simulink model "burckhardt_tire_model"  (R2022b)
settings: Solver=VariableStepAuto  StartTime=0.0  StopTime=10.0  RelTol=1e-3
values from neighbouring files (symbols this model uses):
  Fz = 3000    [burckhardt_model.m]
  road_type = i    [burckhardt_model.m]
undefined symbols (not defined in the file or in its folder): s
settings Model: Creator=FATMANURATA  LastModifiedBy=FATMANURATA

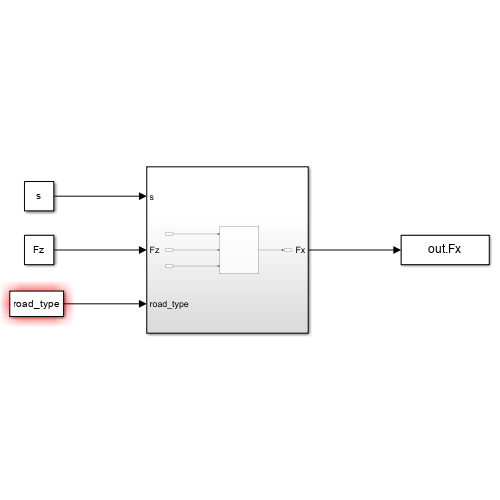
[thumbnail: Simulink's stored preview of the top-level diagram]
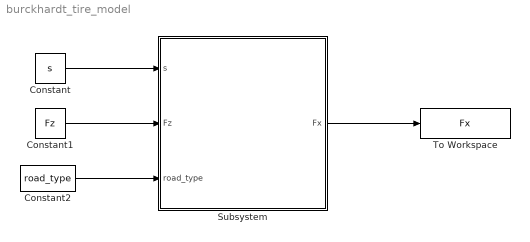
== system burckhardt_tire_model ==
  Constant : Constant  Value=s
  Constant1 : Constant  Value=Fz
  Constant2 : Constant  Value=road_type
  Subsystem : Subsystem
  To Workspace : ToWorkspace  VariableName=Fx  SampleTime=-1
  wires:
  Constant/1 -> Subsystem/1(s)
  Constant1/1 -> Subsystem/2(Fz)
  Constant2/1 -> Subsystem/3(road_type)
  Subsystem/1(Fx) -> To Workspace/1

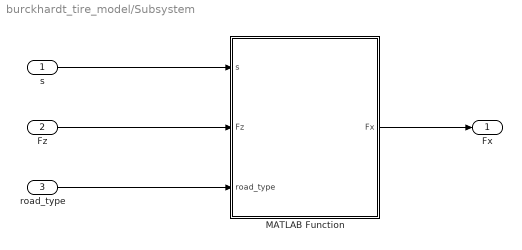
== system burckhardt_tire_model/Subsystem ==
  s : Inport
  Fz : Inport  Port=2
  road_type : Inport  Port=3
  MATLAB Function : MATLAB Function  TreatAsAtomicUnit=on
  Fx : Outport
  wires:
  s/1 -> MATLAB Function/1(s)
  MATLAB Function/1(Fx) -> Fx/1
  Fz/1 -> MATLAB Function/2(Fz)
  road_type/1 -> MATLAB Function/3(road_type)

== matlab function burckhardt_tire_model/Subsystem/MATLAB Function ==
  data: s input; Fx output; Fz input; road_type input
function Fx = fcn(s, Fz, road_type)
   
    % Table:  Burckhardttiremodelparameters.
    

    %      c1       c2        c3
    C = [1.2801, 23.9900, 0.5200;   % 1. Dry Asphalt
         0.8570, 33.8000, 0.3470;   % 2. Wet Asphalt
         1.1973, 25.1680, 0.5373;   % 3. Dry Concrete
         0.1946, 94.1290, 0.0646;   % 4. Snow
         0.0500, 306.3900, 0.0010]; % 5. Ice

    % Geçersiz road_type girişini engellemek için kontrol
    idx = round(road_type);
    if idx < 1 || idx > 5
        idx = 1; % Varsayılan kuru asfalt
    end

    c1 = C(idx, 1);
    c2 = C(idx, 2);
    c3 = C(idx, 3);

    % Burckhardt Formülü
    % mu(s) = c1*(1 - exp(-c2*s)) - c3*s
    % Fx = Fz * mu(s)
    Fx = Fz * (c1 * (1 - exp(-c2 * s)) - c3 * s);
end
